simulink model "LinearCapacitoreModeling"  (R2023a)
settings: Solver=VariableStepAuto  StartTime=0.0  StopTime=0.05  RelTol=1e-3
libraries: fl_lib x8, nesl_utility x5, ee_lib x1
settings Model: Creator=Utente  LastModifiedBy=Utente

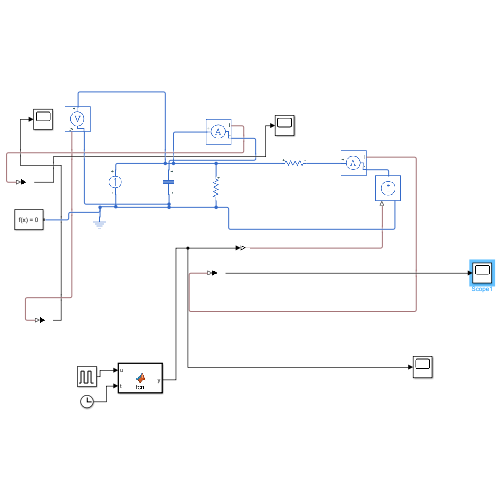
[thumbnail: Simulink's stored preview of the top-level diagram]
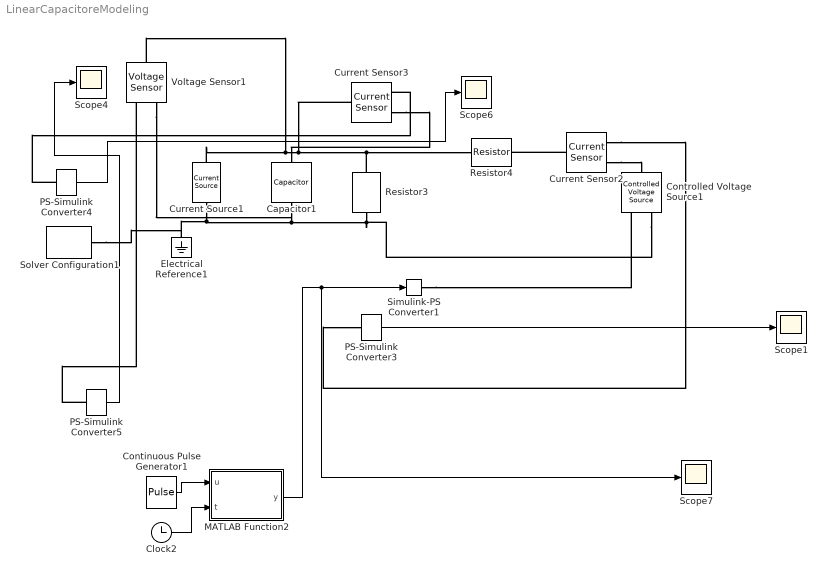
== system LinearCapacitoreModeling ==
  Capacitor1 : fl_lib/Electrical/Electrical Elements/Capacitor  c=0.0037733 F  r=0 Ohm  g=0 1/Ohm  i_specify=on  i_priority=None  i=0 A  i_nominal_specify=off  i_nominal_unit=A  i_nominal_value=1  v_specify=off  v_priority=None  v=0 V  v_nominal_specify=off  v_nominal_unit=V  v_nominal_value=1  vc_specify=off  vc_priority=High  vc=0 V  vc_nominal_specify=off  vc_nominal_unit=V  vc_nominal_value=1
  Clock2 : Clock
  Continuous Pulse Generator1 : DiscretePulseGenerator  PulseType=Time based  Period=3  PulseWidth=50
  Controlled Voltage Source1 : fl_lib/Electrical/Electrical Sources/Controlled Voltage Source
  Current Sensor2 : fl_lib/Electrical/Electrical Sensors/Current Sensor
  Current Sensor3 : fl_lib/Electrical/Electrical Sensors/Current Sensor
  Current Source1 : ee_lib/Sources/Current Source  dc_current=8.09 A  ac_current=0 A  ac_shift=0 rad  ac_frequency=60 Hz  noise_mode=0  PSD=0 A^2/Hz  sample_time=1e-3 s  repeatability=1  user_seed=0  auto_seed=3499211588  i_specify=off  i_priority=None  i=0 A  i_nominal_specify=off  i_nominal_unit=A  i_nominal_value=1  v_specify=off  v_priority=None  v=0 V  v_nominal_specify=off  v_nominal_unit=V  v_nominal_value=1
  Electrical Reference1 : fl_lib/Electrical/Electrical Elements/Electrical Reference
  MATLAB Function2 : MATLAB Function  TreatAsAtomicUnit=on
  PS-Simulink Converter3 : nesl_utility/PS-Simulink Converter  PhysicalDomain=network_engine_domain  SubClassName=ps_output  LeftPortType=input  RightPortType=output  PseudoPeriodic=off  Frequencies=[]  VectorFormat=1-D array  Unit=1  AffineConversion=off
  PS-Simulink Converter4 : nesl_utility/PS-Simulink Converter  PhysicalDomain=network_engine_domain  SubClassName=ps_output  LeftPortType=input  RightPortType=output  PseudoPeriodic=off  Frequencies=[]  VectorFormat=1-D array  Unit=1  AffineConversion=off
  PS-Simulink Converter5 : nesl_utility/PS-Simulink Converter  PhysicalDomain=network_engine_domain  SubClassName=ps_output  LeftPortType=input  RightPortType=output  PseudoPeriodic=off  Frequencies=[]  VectorFormat=1-D array  Unit=1  AffineConversion=off
  Resistor3 : fl_lib/Electrical/Electrical Elements/Resistor  R=93.0571 Ohm  i_specify=off  i_priority=None  i=0 A  i_nominal_specify=off  i_nominal_unit=A  i_nominal_value=1  v_specify=off  v_priority=None  v=0 V  v_nominal_specify=off  v_nominal_unit=V  v_nominal_value=1
  Resistor4 : fl_lib/Electrical/Electrical Elements/Resistor  R=0.2185 Ohm  i_specify=off  i_priority=None  i=0 A  i_nominal_specify=off  i_nominal_unit=A  i_nominal_value=1  v_specify=off  v_priority=None  v=0 V  v_nominal_specify=off  v_nominal_unit=V  v_nominal_value=1
  Scope{1,4,6..7} (4 alike) : Scope
  Simulink-PS Converter1 : nesl_utility/Simulink-PS Converter  PhysicalDomain=network_engine_domain  SubClassName=ps_input  LeftPortType=input  RightPortType=output  PseudoPeriodic=off  Frequencies=[]  NoiseDistribution=none  NoiseParameters=[]  Unit=1  AffineConversion=off  FilteringAndDerivatives=provide  SimscapeFilterOrder=1  InputFilterTimeConstant=0.001  UdotUserProvided=0
  Solver Configuration1 : nesl_utility/Solver Configuration  PhysicalDomain=network_engine_domain  SubClassName=solver  LeftPortType=input  RightPortType=generic  Tones=[]  Harmonics=[]  SimulateNoise=off  Profile=off  UseLocalSampling=off  EnableSwitchedLinearOptims=on  FrequencyDomain=off  UseCCode=off  RelTol=0.001  AbsTol=1e-06  MinStep=1e-09  ToWorkspace=off  RevertToSquareIcSolve=off  NumHomotopyIterations=100  PhasorMode=off  PhasorModeNumHarmonics=1  ConsistencySolver=NEWTON_FTOL  IndexReductionMethod=None  DoDC=on  ResidualTolerance=1e-09  ConsistencyTolSource=GLOBAL  ConsistencyAbsTol=0.001  ConsistencyRelTol=0.001  ConsistencyTolFactor=0.001  UseLocalSolver=off  LocalSolverChoice=NE_BACKWARD_EULER_ADVANCER  ResolveIndetEquations=on  FunctionEvalNumThread=1  LocalSolverSampleTime=0.001  DoFixedCost=off  MaxNonlinIter=3  MaxModeIter=2  ComputeImpulses=on  ImpulseIterations=2  LinearAlgebra=auto  LinearAlgebraNumThread=0  EquationFormulation=NE_TIME_EF  DelaysMemoryBudget=1024  AutomaticFiltering=on  FilteringTimeConstant=0.001  PartitionStorageMethod=AS_NEEDED  PartitionMemoryBudget=1024  PartitionMethod=ROBUST
  Voltage Sensor1 : fl_lib/Electrical/Electrical Sensors/Voltage Sensor
  wires:
  Continuous Pulse Generator1/1 -> MATLAB Function2/1(u)
  MATLAB Function2/1(y) -> Scope7/1, Simulink-PS Converter1/1
  PS-Simulink Converter3/1 -> Scope1/1
  PS-Simulink Converter4/1 -> Scope6/1
  Clock2/1 -> MATLAB Function2/2(t)
  PS-Simulink Converter5/1 -> Scope4/1
  connections:
  Resistor3/RConn1 -- Electrical Reference1/LConn1 -- Solver Configuration1/RConn1 -- Current Source1/RConn1 -- Voltage Sensor1/RConn2 -- Capacitor1/RConn1 -- Controlled Voltage Source1/RConn2
  Voltage Sensor1/LConn1 -- Current Source1/LConn1 -- Current Sensor3/LConn1 -- Resistor3/LConn1 -- Resistor4/LConn1
  Current Sensor2/RConn2 -- Controlled Voltage Source1/LConn1
  Current Sensor2/LConn1 -- Resistor4/RConn1
  PS-Simulink Converter4/LConn1 -- Current Sensor3/RConn1
  PS-Simulink Converter5/LConn1 -- Voltage Sensor1/RConn1
  Current Sensor3/RConn2 -- Capacitor1/LConn1
  Simulink-PS Converter1/RConn1 -- Controlled Voltage Source1/RConn1
  Current Sensor2/RConn1 -- PS-Simulink Converter3/LConn1

== matlab function LinearCapacitoreModeling/MATLAB Function2 ==
  data: u input; y output; t input
function y = fcn(u, t)
    % Define voltage levels
    V1 = 23.2; % First level
    V2 = 23.4; % Second level
    V3 = 23.6; % Third level
    V4 = 23.4; % Fourth level
    V5 = 23.2; % Final level

    % Define step times in milliseconds
    T1 = 0.01; % Time for V1 to V2 (10 milliseconds)
    T2 = 0.02; % Time for V2 to V3 (20 milliseconds)
    T3 = 0.03; % Time for V3 to V4 (30 milliseconds)
    T4 = 0.04; % Time for V4 to V5 (40 milliseconds)

    % Define transition time for smooth change
    transition_time = 0; % 3 milliseconds for smooth transition

    % Repeat every 40 milliseconds
    t_mod = mod(t, T4); % Modulo time to repeat every 40 milliseconds

    % Logic to generate the stepped waveform with smooth transitions
    if t_mod < T1 - transition_time
        y = V1;
    elseif t_mod < T1
        % Smooth transition from V1 to V2
        y = V1 + (V2 - V1) * ((t_mod - (T1 - transition_time)) / transition_time);
    elseif t_mod < T2 - transition_time
        y = V2;
    elseif t_mod < T2
        % Smooth transition from V2 to V3
        y = V2 + (V3 - V2) * ((t_mod - (T2 - transition_time)) / transition_time);
    elseif t_mod < T3 - transition_time
        y = V3;
    elseif t_mod < T3
        % Smooth transition from V3 to V4
        y = V3 + (V4 - V3) * ((t_mod - (T3 - transition_time)) / transition_time);
    elseif t_mod < T4 - transition_time
        y = V4;
    elseif t_mod < T4
        % Smooth transition from V4 to V5
        y = V4 + (V5 - V4) * ((t_mod - (T4 - transition_time)) / transition_time);
    else
        y = V5;
    end
end
